simulink model "lab1"  (R2021a)
settings: Solver=VariableStepAuto  StartTime=0.0  StopTime=1.00  RelTol=1e-3
libraries: fuzblock x1, simulink x1
settings Model: Creator=toe75  LastModifiedBy=toe75

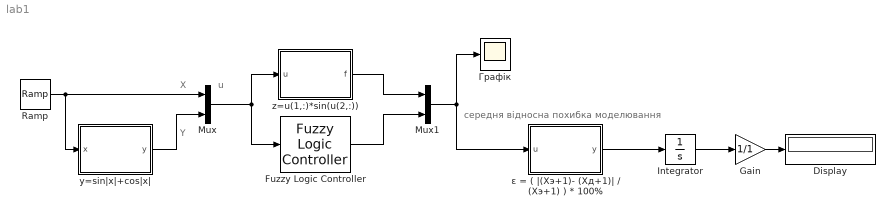
== system lab1 ==
  note: u
  note: Y
  note: X
  note: середня відносна похибка моделювання
  Display : Display
  Fuzzy Logic Controller : fuzblock/Fuzzy Logic  Controller  FIS='lab1_gaus.fis'  OutputSampleNumber=101  DataType=double  FuzzifiedInputs=off  RuleFiringStrengths=off  RuleOutputs=off  AggregatedOutputs=off  SimulateUsing=Interpreted execution  OutOfRangeInputValueMessage=warning  NoRuleFiredMessage=warning  EmptyOutputFuzzySetMessage=warning
  Gain : Gain  Gain=1/1
  Integrator : Integrator
  Mux : Mux  Inputs=2
  Mux1 : Mux  Inputs=2
  Ramp : simulink/Sources/Ramp  slope=1  start=0  InitialOutput=0
  y=sin|x|+cos|x| : MATLAB Function  TreatAsAtomicUnit=on
  z=u(1,:)*sin(u(2,:)) : MATLAB Function  TreatAsAtomicUnit=on
  ε = ( |(Хэ+1)- (Хд+1)| / (Хэ+1) ) * 100% : MATLAB Function  TreatAsAtomicUnit=on
  Графiк : Scope
  wires:
  Ramp/1 -> Mux/1, y=sin|x|+cos|x|/1(x)
  y=sin|x|+cos|x|/1(y) -> Mux/2
  Mux/1 -> Fuzzy Logic Controller/1, z=u(1,:)*sin(u(2,:))/1(u)
  z=u(1,:)*sin(u(2,:))/1(f) -> Mux1/1
  Fuzzy Logic Controller/1 -> Mux1/2
  Mux1/1 -> Графiк/1, ε = ( |(Хэ+1)- (Хд+1)| / (Хэ+1) ) * 100%/1(u)
  ε = ( |(Хэ+1)- (Хд+1)| / (Хэ+1) ) * 100%/1(y) -> Integrator/1
  Integrator/1 -> Gain/1
  Gain/1 -> Display/1

== matlab function lab1/y=sin|x|+cos|x| ==
  data: x input; y output
function y = fcn(x)
y = sin(abs(x))+ cos(abs(x));

== matlab function lab1/ε = ( |(Хэ+1)- (Хд+1)| // (Хэ+1) ) * 100% ==
  data: u input; y output
function y = fcn(u)
y = (abs(u(1,:)-u(2,:)))/(u(1,:)+1)*100;

== matlab function lab1/z=u(1,:)*sin(u(2,:)) ==
  data: u input; f output
function f = fcn(u)
f = u(1,:)*sin(u(2,:));
